simulink model "simulation_mpc"  (R2021b)
settings: Solver=FixedStepAuto  StartTime=0.0  StopTime=T  RelTol=1e-3  EnableMultiTasking=on
undefined symbols (not defined in the file or in its folder): discrete_0, h, Humusoft, MF634
libraries: sldrtlib x2, eeLuenbergerObserver x1, mpclib x1, quarc_library x1, simulink x1
settings Model: Creator=rbabuska  LastModifiedBy=wilbe
settings SolverCC: AlgebraicLoopSolver=TrustRegion  AutoInsertRateTranBlk=on
settings DataIOCC: LimitDataPoints=on  SaveFormat=Array  SignalLoggingSaveFormat=ModelDataLogs  SaveOutput=off  SaveTime=off  ReturnWorkspaceOutputs=off
settings OptimizationCC: DefaultParameterBehavior=Inlined  InlineInvariantSignals=on  EnhancedBackFolding=on  PassReuseOutputArgsAs=Individual arguments  ExpressionDepthLimit=2147483647  StateBitsets=on  DataBitsets=on  ZeroExternalMemoryAtStartup=off  ZeroInternalMemoryAtStartup=off  NoFixptDivByZeroProtection=on  LifeSpan=1  OptimizeBlockOrder=speed  DifferentSizesBufferReuse=on  EfficientTunableParamExpr=on
settings DebuggingCC: UnderspecifiedInitializationDetection=Classic  MergeDetectMultiDrivingBlocksExec=none  ParameterTunabilityLossMsg=error  FcnCallInpInsideContextMsg=warning  StateNameClashWarn=warning  SFUnexpectedBacktrackingDiag=warning  SFNoUnconditionalDefaultTransitionDiag=warning  SFExecutionAtInitializationDiag=none  SFMachineParentedDataDiag=warning  ArithmeticOperatorsInVariantConditions=warning
settings HardwareCC: ProdBitPerPointer=32  ProdBitPerSizeT=32  ProdBitPerPtrDiffT=32  ProdLargestAtomicFloat=None  ProdIntDivRoundTo=Floor  ProdWordSize=32  ProdHWDeviceType=Generic->Custom
settings ModelReferenceCC: PropagateSignalLabelsOutOfModel=off
settings SFSimCC: SimUseLocalCustomCode=off  MATLABDynamicMemAlloc=off  CustomCodeUndefinedFunction=UseInterfaceOnly
settings RTWCC: Description=Embedded Coder  SystemTargetFile=ert.tlc  TLCOptions=-p0  GenCodeOnly=on  TemplateMakefile=ert_default_tmf  GenerateReport=on  RTWVerbose=off  RTWUseLocalCustomCode=off  IncludeHyperlinkInReport=on  LaunchReport=on
settings CodeAppCC: ForceParamTrailComments=on  IgnoreCustomStorageClasses=off  OperatorAnnotations=on  SimulinkDataObjDesc=on  SFDataObjDesc=on  CustomSymbolStrGlobalVar=rt$N$M  CustomSymbolStrType=$N$M  CustomSymbolStrFcn=$N$M$F  CustomSymbolStrMacro=$N$M  InsertBlockDesc=on
settings ERTTargetCC: CodeReplacementLibrary=ISO_C  GenerateSampleERTMain=on  IncludeMdlTerminateFcn=off  SuppressErrorStatus=on  SupportAbsoluteTime=off  PurelyIntegerCode=on  SupportNonFinite=off  SupportComplex=off  InlinedParameterPlacement=NonHierarchical  RootIOFormat=Structure reference  ERTCustomFileTemplate=example_file_process.tlc
settings ConfigComp: CovMetricSettings=dw  CovSaveCumulativeToWorkspaceVar=on  CovSaveSingleToWorkspaceVar=on  CovExternalEMLEnable=off  CovSFcnEnable=off

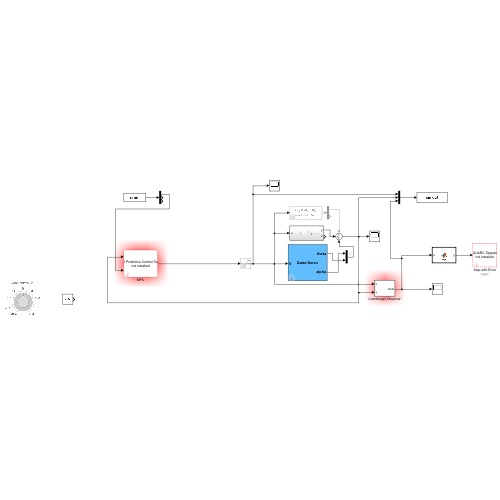
[thumbnail: Simulink's stored preview of the top-level diagram]
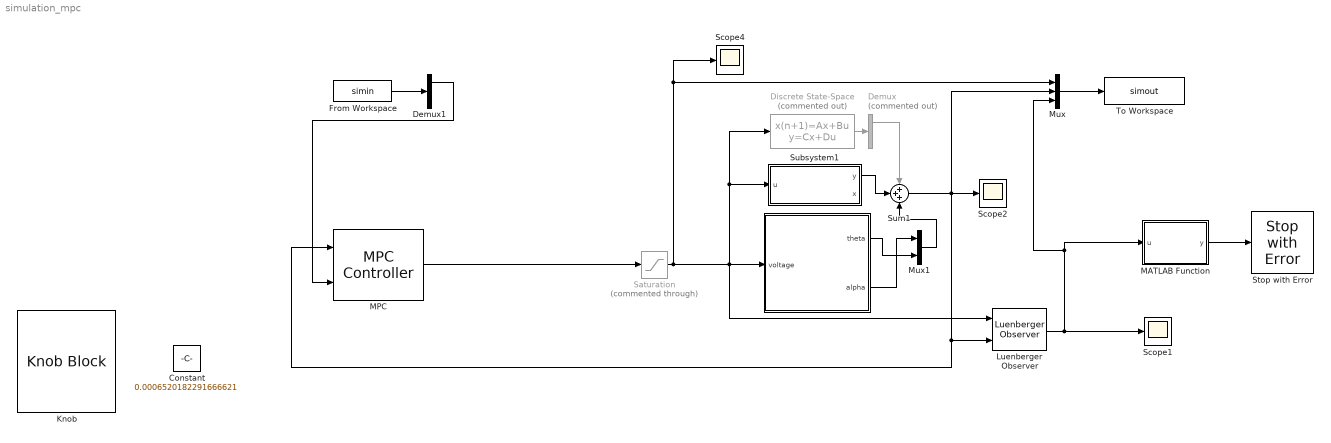
== system simulation_mpc ==
  " " : Subsystem  LoadFcn=hwinit  InitFcn=hwinit  mask{h=h}
      mask prompts: h "Sampling period [s]"
      mask Display:
      | disp('Qube-Servo')
      | port_label('output',1,'theta')
      | port_label('output',2,'alpha')
      | port_label('input',1,'V')
  Constant : Constant  Value=0.0006520182291666621
  Demux : Demux  Commented=on  Outputs=[2;4]
  Demux1 : Demux  Outputs=3
  Discrete State-Space : DiscreteStateSpace  Commented=on  A=discrete_0.A  B=discrete_0.B  C=[discrete_0.C;eye(4)]  D=[discrete_0.D;zeros(4,1)]  InitialCondition=[0;0;0;0]  SampleTime=h
  From Workspace : FromWorkspace  VariableName=simin  SampleTime=h  OutputAfterFinalValue=Holding final value
  Knob : KnobBlock  ScaleMin=-0.4  ScaleMax=0.4
  Luenberger Observer : eeLuenbergerObserver/Luenberger Observer  StateSpaceType=Discrete-time  Ad=discrete_0.A  Bd=discrete_0.B  Cd=discrete_0.C  Dd=discrete_0.D  A=1  B=1  C=1  D=1  ObserverDesign=Observer gain  Ld=disc  DesiredEigenvalues=pDisc  x0=[0;0;0;0]  Tsd=0.1  Ts=h
      settings: SourceProductBaseCode=PS
  MATLAB Function : MATLAB Function  TreatAsAtomicUnit=on
  MPC : mpclib/MPC Controller  SCDEnableBlockLinearizationSpecification=on  mpcobj=mpc1_1_C  is_multiple=0  enable_value=0  return_u0=off  updateMPCinCallerWorkspace=on  md_inport=off  mv_inport=off  uref_inport=off  return_cost=off  return_mvseq=off  return_qpstatus=off  return_xseq=off  return_state=off  return_ovseq=off  state_inport=off  umin_inport=off  umax_inport=off  ymin_inport=off  ymax_inport=off  cc_inport=off  ywt_inport=off  uwt_inport=off  duwt_inport=off  rhoeps_inport=off  pm_inport=off  MaximumP=10  HorizonChoice=FixedHorizon  n_ts=0.005  n_p=50  n_mv=1  n_md=0  n_ud=0  n_mo=2  n_uo=0  BlockDataType=double  SampleTimeInherited=off  switch_inport=off
  Mux : Mux  Inputs=3
  Mux1 : Mux  Inputs=2
  Saturation : Saturate  Commented=through  UpperLimit=0.2  LowerLimit=-0.2
  Scope1 : Scope
  Scope2 : Scope
  Scope4 : Scope
  Stop with Error : quarc_library/Sinks/Error Handling/Stop with Error  message_type=Fixed error message  message=Error occurred
      settings: AttributesFormatString="\"%<message>\""  SourceProductName=QUARC Targets
  Subsystem1 : Subsystem
  Sum1 : Sum  Inputs=+++
  To Workspace : ToWorkspace  VariableName=simout  SaveFormat=Timeseries  SampleTime=-1
  wires:
  Mux/1 -> To Workspace/1
  Luenberger Observer/1 -> MATLAB Function/1(u), Mux/3, Scope1/1
  Discrete State-Space/1 -> Demux/1
  Saturation/1 -> " "/1(voltage), Luenberger Observer/1, Subsystem1/1(u), Discrete State-Space/1, Scope4/1, Mux/1
  " "/2(alpha) -> Mux1/1
  " "/1(theta) -> Mux1/2
  Subsystem1/1(y) -> Sum1/2
  Demux/1 -> Sum1/1
  From Workspace/1 -> Demux1/1
  Demux1/1 -> MPC/2
  Mux1/1 -> Sum1/3
  MPC/1 -> Saturation/1
  Sum1/1 -> MPC/1, Luenberger Observer/2, Scope2/1, Mux/2
  MATLAB Function/1(y) -> Stop with Error/1

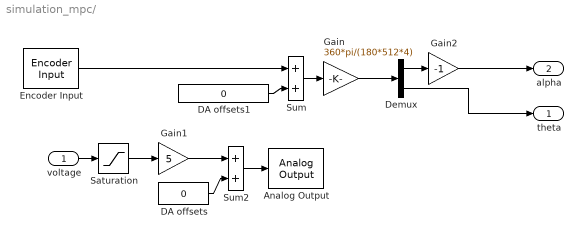
== system simulation_mpc/  ==
  voltage : Inport
  Analog Output : sldrtlib/Analog Output  SampleTime=h  MaxMissedTicks=100  ShowMissedTicks=off  YieldWhenWaiting=off  DrvName=Humusoft/MF634  DrvAddress=4294967295  DrvOptions=0  Channels=[1]  RangeMode=2  VoltRange=1  InitialValue=0  FinalValue=0
      settings: AttributesFormatString=Humusoft\nMF634 [auto]
  DA offsets : Constant  Value=0
  DA offsets1 : Constant  Value=0  SampleTime=h
  Demux : Demux  Outputs=2
  Encoder Input : sldrtlib/Encoder Input  SampleTime=h  MaxMissedTicks=100  ShowMissedTicks=off  YieldWhenWaiting=off  DrvName=Humusoft/MF634  DrvAddress=4294967295  DrvOptions=0  Channels=[1,2]  QuadMode=3  IndexPulse=1  InputFilter=Inf  DataType=1
      settings: AttributesFormatString=Humusoft\nMF634 [auto]
  Gain : Gain  Gain=360*pi/(180*512*4)  SaturateOnIntegerOverflow=on  OutDataTypeStr=Inherit: Same as input  ParamDataTypeStr=Inherit: Same as input
  Gain1 : Gain  Gain=5  SaturateOnIntegerOverflow=on  OutDataTypeStr=Inherit: Same as input  ParamDataTypeStr=Inherit: Same as input
  Gain2 : Gain  Gain=-1  SaturateOnIntegerOverflow=on  OutDataTypeStr=Inherit: Same as input  ParamDataTypeStr=Inherit: Same as input
  Saturation : Saturate  UpperLimit=1  LowerLimit=-1
  Sum : Sum  InputSameDT=on  SaturateOnIntegerOverflow=on  OutDataTypeStr=Inherit: Same as first input
  Sum2 : Sum  InputSameDT=on  SaturateOnIntegerOverflow=on  OutDataTypeStr=Inherit: Same as first input
  theta : Outport  Tag=Cable length
  alpha : Outport  Tag=Cable length  Port=2
  wires:
  Sum/1 -> Gain/1
  DA offsets1/1 -> Sum/2
  Gain1/1 -> Sum2/1
  Sum2/1 -> Analog Output/1
  DA offsets/1 -> Sum2/2
  voltage/1 -> Saturation/1
  Encoder Input/1 -> Sum/1
  Saturation/1 -> Gain1/1
  Demux/1 -> Gain2/1
  Gain/1 -> Demux/1
  Gain2/1 -> alpha/1
  Demux/2 -> theta/1

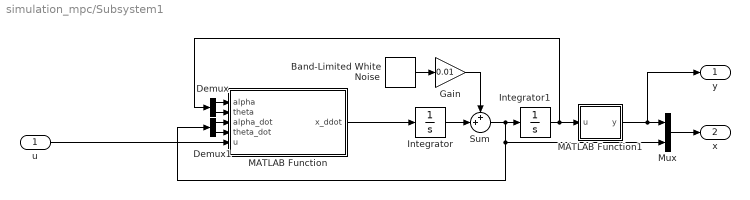
== system simulation_mpc/Subsystem1 ==
  u : Inport
  Band-Limited White Noise : simulink/Sources/Band-Limited White Noise  Cov=1  Ts=h  seed=[23341]
  Demux : Demux  Outputs=2
  Demux1 : Demux  Outputs=2
  Gain : Gain  Gain=0.01
  Integrator : Integrator
  Integrator1 : Integrator  InitialCondition=[0;pi]
  MATLAB Function : MATLAB Function  TreatAsAtomicUnit=on
  MATLAB Function1 : MATLAB Function  TreatAsAtomicUnit=on
  Mux : Mux  Inputs=2
  Sum : Sum  Inputs=++|
  y : Outport  PortDimensions=2
  x : Outport  Port=2  PortDimensions=4
  wires:
  Integrator/1 -> Sum/2
  Sum/1 -> Mux/2, Demux1/1, Integrator1/1
  Demux/2 -> MATLAB Function/2(theta)
  Demux/1 -> MATLAB Function/1(alpha)
  MATLAB Function1/1(y) -> y/1, Mux/1
  MATLAB Function/1(x_ddot) -> Integrator/1
  Demux1/2 -> MATLAB Function/4(theta_dot)
  Demux1/1 -> MATLAB Function/3(alpha_dot)
  u/1 -> MATLAB Function/5(u)
  Mux/1 -> x/1
  Band-Limited White Noise/1 -> Gain/1
  Gain/1 -> Sum/1
  Integrator1/1 -> MATLAB Function1/1(u), Demux/1

== matlab function simulation_mpc/MATLAB Function ==
  data: u input; y output
function y = fcn(u)
neartop=abs(u(2))<45/180*pi;%10deg from top
% slowtheta=abs(u(4))<30/180*pi;%10deg/sec
y=~neartop;

== matlab function simulation_mpc/Subsystem1/MATLAB Function ==
  data: alpha input; theta input; alpha_dot input; theta_dot input; x_ddot output; u input
function x_ddot = generated_nonlinfit(alpha,theta,alpha_dot,theta_dot,u)
%GENERATED_NONLINFIT
%    X_DDOT = GENERATED_NONLINFIT(ALPHA,THETA,ALPHA_DOT,THETA_DOT,U)

%    This function was generated by the Symbolic Math Toolbox version 9.0.
%    20-Oct-2022 11:58:04

t2 = cos(theta);
t3 = sin(theta);
t4 = theta_dot.^2;
t5 = t2.^2;
t6 = t5.*5.202e-4;
t7 = t6-1.033684280825389e-3;
t8 = 1.0./t7;
et1 = alpha.*(-1.114482127011352e-2)-alpha_dot.*1.457479237134593e-3+u.*5.145679542825577e-1;
et2 = t2.*t3.*4.388810825838219e-2+t3.*t4.*3.668526888060489e-4+t2.*theta_dot.*3.637246567579307e-5;
et3 = t3.*8.895381886637765e-5;
et4 = theta_dot.*7.372087455672215e-8-alpha.*t2.*1.136771769551579e-5;
et5 = alpha_dot.*t2.*(-1.486628821877285e-6)+t2.*u.*5.248593133682088e-4+t2.*t3.*t4.*3.741897425821699e-7;
x_ddot = [t8.*(et1+et2).*(-1.367960533786131);t8.*(et3+et4+et5).*1.390203794498101e+3];

== matlab function simulation_mpc/Subsystem1/MATLAB Function1 ==
  data: u input; y output
function y = wrap(u)
y=[
    u(1)
    wrapToPi(u(2)-pi)
];
